simulink model "MSDCtrl"  (R2024b)
settings: Solver=VariableStepAuto  StartTime=0.0  StopTime=10.0  RelTol=1e-3
settings Model: Creator=Robin  LastModifiedBy=Robin

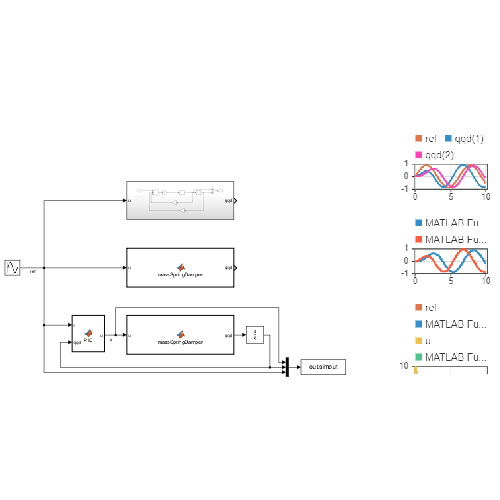
[thumbnail: Simulink's stored preview of the top-level diagram]
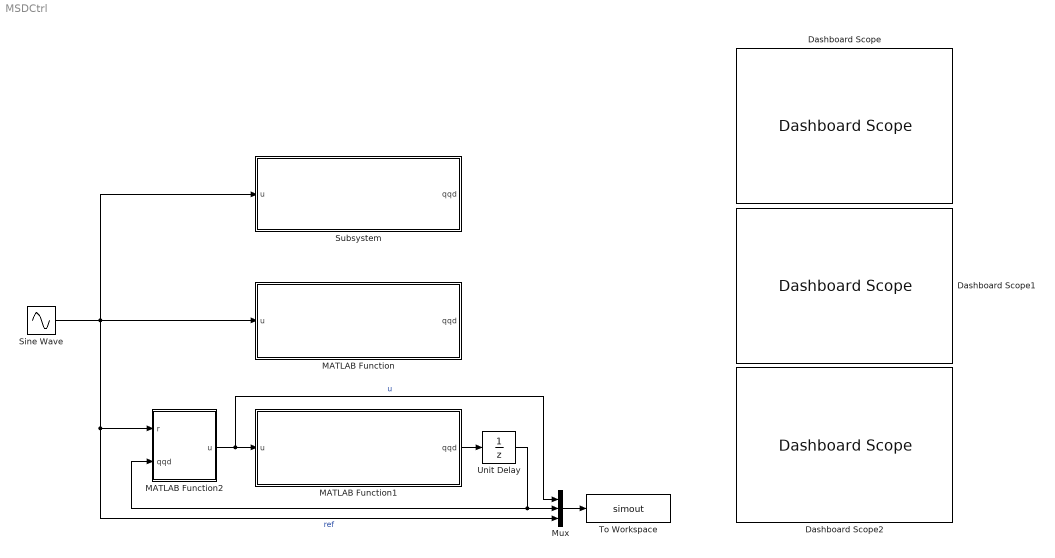
== system MSDCtrl ==
  Dashboard Scope : DashboardScope
  Dashboard Scope1 : DashboardScope
  Dashboard Scope2 : DashboardScope
  MATLAB Function : MATLAB Function  TreatAsAtomicUnit=on  SystemSampleTime=0.01
  MATLAB Function1 : MATLAB Function  TreatAsAtomicUnit=on  SystemSampleTime=0.01
  MATLAB Function2 : MATLAB Function  TreatAsAtomicUnit=on
  Mux : Mux  Inputs=3
  Sine Wave : Sin  SampleTime=0
  Subsystem : Subsystem
  To Workspace : ToWorkspace  VariableName=simout  SaveFormat=Timeseries  SampleTime=-1
  Unit Delay : UnitDelay  SampleTime=-1  HasFrameUpgradeWarning=on
  wires:
  Sine Wave/1 -> Mux/3, MATLAB Function2/1(r), Subsystem/1(u), MATLAB Function/1(u)  "ref"
  MATLAB Function2/1(u) -> Mux/1, MATLAB Function1/1(u)  "u"
  MATLAB Function1/1(qqd) -> Unit Delay/1
  Unit Delay/1 -> Mux/2, MATLAB Function2/2(qqd)
  Mux/1 -> To Workspace/1

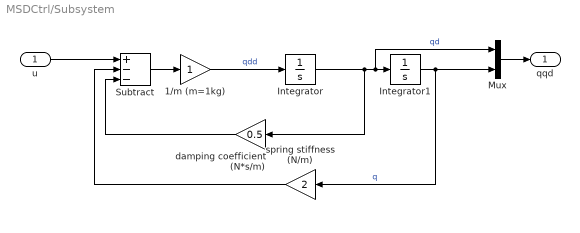
== system MSDCtrl/Subsystem ==
  u : Inport
  1/m (m=1kg) : Gain
  Integrator : Integrator
  Integrator1 : Integrator
  Mux : Mux  Inputs=2
  Subtract : Sum  Inputs=+--
  damping coefficient (N*s/m) : Gain  Gain=0.5
  spring stiffness (N/m) : Gain  Gain=2
  qqd : Outport
  wires:
  u/1 -> Subtract/1
  1/m (m=1kg)/1 -> Integrator/1  "qdd"
  Subtract/1 -> 1/m (m=1kg)/1
  Integrator/1 -> damping coefficient (N*s/m)/1, Mux/1, Integrator1/1  "qd"
  Integrator1/1 -> Mux/2, spring stiffness (N/m)/1  "q"
  damping coefficient (N*s/m)/1 -> Subtract/3
  spring stiffness (N/m)/1 -> Subtract/2
  Mux/1 -> qqd/1

== matlab function MSDCtrl/MATLAB Function ==
  settings: updateMethod=DISCRETE
  data: u input; qqd output
function qqd = massSpringDamper(u)
% Continuous-time mass-spring-damper system
% u: input force (N)
% pos: output position (m)
% vel: output velocity (m/s)

%% system paramters
m = 1.0;    % Mass (kg
c = 0.5;    % Damping coefficient (Ns/m)
k = 2.0;    % Spring stiffness (N/m)
Ts = 0.01;  % Sample time(s)

%% Persistent state variables
persistent q_prev
if isempty(q_prev)
    q_prev = [0, 0]; % Initial condition [position, velocity]
end

%% Compute acceleration
qdd = (u - c * q_prev(2) - k * q_prev(1)) / m;

%% update states using Euler integration
qd = q_prev(2) + Ts * qdd;
q = q_prev(1) + Ts * qd;

%% Update persistent variables
q_prev = [q, qd];

%% Output;
qqd = q_prev;

== matlab function MSDCtrl/MATLAB Function2 ==
  settings: updateMethod=DISCRETE
  data: r input; u output; qqd input
function u = PID(r, qqd)
% Determine control action from proportional, integral and derivatibe gains

%% Sample Time
Ts = 0.01;  %(s)

%% Gains constants
Kp = 100; % Proportional gain
Ki = 10; % Integral gain
Kd = 10; % Derivative gain

%% Persitent error
persistent integral_error prev_error
if isempty(integral_error)
    integral_error = 0;
    prev_error = 0;
end

%% Compute errors
proportional_error = r - qqd(1);
integral_error = integral_error + proportional_error *Ts;
derivative_error = (proportional_error - prev_error)/Ts;

%% Control law
u = Kp * proportional_error + Ki * integral_error + Kd * derivative_error;

%% Saturation;
u = max(min(u,10), -10);

%% Update persitent state
prev_error = proportional_error;

== matlab function MSDCtrl/MATLAB Function1 ==
  settings: updateMethod=DISCRETE
  data: u input; qqd output
function qqd = massSpringDamper(u)
% Continuous-time mass-spring-damper system
% u: input force (N)
% pos: output position (m)
% vel: output velocity (m/s)

%% system paramters
m = 1.0;    % Mass (kg
c = 0.5;    % Damping coefficient (Ns/m)
k = 2.0;    % Spring stiffness (N/m)
Ts = 0.01;  % Sample time(s)

%% Persistent state variables
persistent q_prev
if isempty(q_prev)
    q_prev = [0, 0]; % Initial condition [position, velocity]
end

%% Compute acceleration
qdd = (u - c * q_prev(2) - k * q_prev(1)) / m;

%% update states using Euler integration
qd = q_prev(2) + Ts * qdd;
q = q_prev(1) + Ts * qd;

%% Update persistent variables
q_prev = [q, qd];

%% Output;
qqd = q_prev;
